simulink model "four_1"  (R2018a)
settings: Solver=ode23tb  StartTime=0.0  StopTime=0.1  RelTol=1e-3
libraries: powerlib x15, powerlib_extras x1
settings Model: Creator=14064  LastModifiedBy=14064

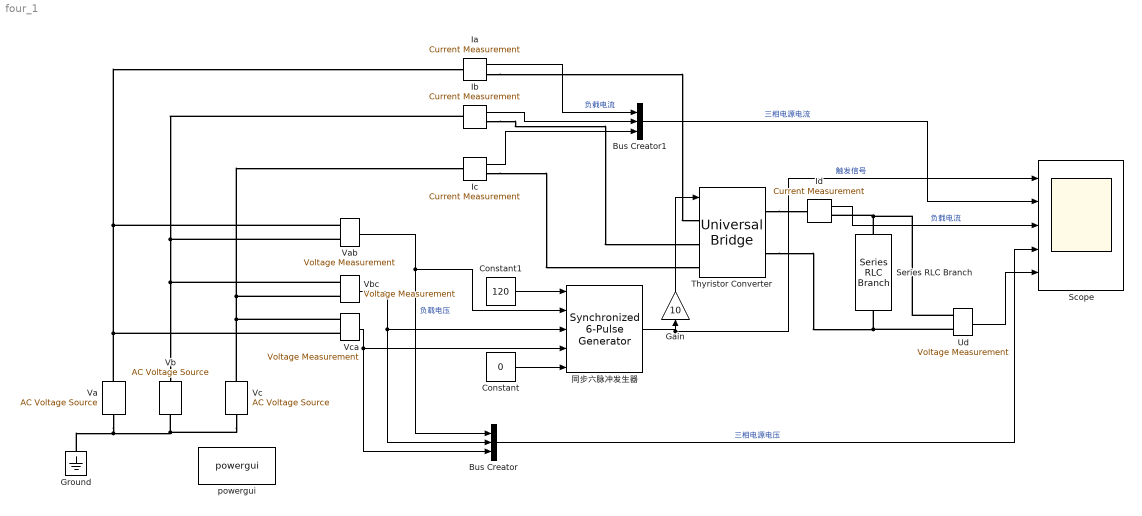
== system four_1 ==
  Bus Creator : BusCreator  Inputs=3
  Bus Creator1 : BusCreator  Inputs=3
  Constant : Constant  Value=0
  Constant1 : Constant  Value=120
  Gain : Gain  Gain=10
  Ground : powerlib/Elements/Ground  LConnTagsString=a
  Ia : powerlib/Measurements/Current Measurement  PhasorSimulation=off  OutputType=Complex  PSBequivalent=0
  Ib : powerlib/Measurements/Current Measurement  PhasorSimulation=off  OutputType=Complex  PSBequivalent=0
  Ic : powerlib/Measurements/Current Measurement  PhasorSimulation=off  OutputType=Complex  PSBequivalent=0
  Id : powerlib/Measurements/Current Measurement  PhasorSimulation=off  OutputType=Complex  PSBequivalent=0
  Scope : Scope  NumInputPorts=5
  Series RLC Branch : powerlib/Elements/Series RLC Branch  LConnTagsString=__new0  RConnTagsString=__new0  BranchType=R  Resistance=5  Inductance=0.7  SetiL0=off  InitialCurrent=0  Capacitance=inf  Setx0=off  InitialVoltage=0  Measurements=None
  Thyristor Converter : powerlib/Power Electronics/Universal Bridge  Arms=3  SnubberResistance=1e5  SnubberCapacitance=inf  Device=Thyristors  Ron=1e-3  Lon=0  ForwardVoltages="[  0.8  0.8  ]"  ForwardVoltage=0  GTOparameters=[ 10e-6 , 20e-6 ]  IGBTparameters=[ 1e-6 , 2e-6 ]  Measurements=All voltages and currents  Measurements_2=None  converterType=Rectifier
  Ud : powerlib/Measurements/Voltage Measurement  PhasorSimulation=off  OutputType=Complex  PSBequivalent=0
  Va : powerlib/Electrical Sources/AC Voltage Source  Amplitude=380  Phase=0  Frequency=50  SampleTime=0  Measurements=None  BusType=swing  Pref=10e3  Qref=0  Qmin=-inf  Qmax=+inf
  Vab : powerlib/Measurements/Voltage Measurement  PhasorSimulation=off  OutputType=Complex  PSBequivalent=0
  Vb : powerlib/Electrical Sources/AC Voltage Source  Amplitude=380  Phase=-120  Frequency=50  SampleTime=0  Measurements=None  BusType=swing  Pref=10e3  Qref=0  Qmin=-inf  Qmax=+inf
  Vbc : powerlib/Measurements/Voltage Measurement  PhasorSimulation=off  OutputType=Complex  PSBequivalent=0
  Vc : powerlib/Electrical Sources/AC Voltage Source  Amplitude=380  Phase=-240  Frequency=50  SampleTime=0  Measurements=None  BusType=swing  Pref=10e3  Qref=0  Qmin=-inf  Qmax=+inf
  Vca : powerlib/Measurements/Voltage Measurement  PhasorSimulation=off  OutputType=Complex  PSBequivalent=0
  powergui : powerlib/powergui  Priority=1  SimulationMode=Continuous  SampleTime=50e-6  frequency=60  Iterations=50  frequencyindice=50  Pbase=100e6  ErrMax=1e-4  UnitsV=kV  UnitsW=MW  buscounter=0  FunctionMessages=off  echomessages=off  EnableUseOfTLC=off  CurrentSourceSwitches=off  DisableSnubberDevices=off  DisableRonSwitches=off  DisableVfSwitches=off  DisplayEquations=off  SolverType=Tustin/Backward Euler (TBE)  Interpol=off  ExternalGateDelay=off  methode=off  Ts=100  x0status=blocks  SPID=on  SwTol=0  HookPort=off  RestoreLinks=warning  ResistiveCurrentMeasurement=off  Frange=[0:2:500]  Ylog=off  Xlog=on  ShowGrid=off  save=off  variable=ZData  structure=0  ZoomFFT=off  StartTime=0.0  cycles=1  DisplayStyle=1  fundamental=60  FreqAxis=off  MaxFrequency=1000  frequencyindicesteady=1  RmsSteady=1  display=off
  同步六脉冲发生器 : powerlib_extras/Control  Blocks/Synchronized 6-Pulse Generator  freq=60  pwidth=10  Double_Pulse=off
  wires:
  Vab/1 -> 同步六脉冲发生器/2, Bus Creator/1  "负载电压"
  Vbc/1 -> 同步六脉冲发生器/3, Bus Creator/2
  Vca/1 -> 同步六脉冲发生器/4, Bus Creator/3
  Constant/1 -> 同步六脉冲发生器/5
  Constant1/1 -> 同步六脉冲发生器/1
  Ia/1 -> Bus Creator1/1  "负载电流"
  Ib/1 -> Bus Creator1/2
  Ic/1 -> Bus Creator1/3
  Ud/1 -> Scope/5
  同步六脉冲发生器/1 -> Scope/1, Gain/1  "触发信号"
  Gain/1 -> Thyristor Converter/1
  Bus Creator/1 -> Scope/4  "三相电源电压"
  Bus Creator1/1 -> Scope/2  "三相电源电流"
  Id/1 -> Scope/3  "负载电流"
  connections:
  Ground/LConn1 -- Va/LConn1 -- Vc/LConn1 -- Vb/LConn1
  Va/RConn1 -- Vca/LConn2 -- Vab/LConn1 -- Ia/LConn1
  Ib/LConn1 -- Vab/LConn2 -- Vbc/LConn1 -- Vb/RConn1
  Vc/RConn1 -- Vca/LConn1 -- Vbc/LConn2 -- Ic/LConn1
  Ia/RConn1 -- Thyristor Converter/LConn1
  Ib/RConn1 -- Thyristor Converter/LConn2
  Ic/RConn1 -- Thyristor Converter/LConn3
  Thyristor Converter/RConn1 -- Id/LConn1
  Ud/LConn2 -- Thyristor Converter/RConn2 -- Series RLC Branch/RConn1
  Series RLC Branch/LConn1 -- Ud/LConn1 -- Id/RConn1
